simulink library "motohawk_engine_motoshare_lib"  (Simulink 6.3)
undefined symbols (not defined in the file or in its folder): cast_val, IndPowerMax, lookup_group, motohawk_tex, motohawk_vardec_config_group, motohawk_vardec_path, SampleTime, SteadyStateECT, txtTitle, WarmUpTimeConst
libraries: MotoHawk_lib x211, motohawk_control_primitives_lib x20, motohawk_annotations_lib x7, motohawk_engine_lib x5, AutoDoc_lib x4, motohawk_control_primitives_lib_new x3, motohawk_control_primitives_motoshare_lib x2
(part 2 of 7)

== system motohawk_engine_motoshare_lib/Discrete Actuator Characterization ==
  EngUnits : Inport
  0 = No Inversion 1 = Inversion : MotoHawk_lib/Calibration & Probing Blocks/motohawk_calibration  nam=[prefix '_Polarity']  val=boolean(polarity-1)  storage=Calibration  show_more=on  name_source=Use Parameter  data_type=Inherit from 'Default Value'  read_level=1  write_level=1  ovr_cals=on  view_as=Number  enum_struct={'Disabled', 'Enabled'}  vector_style=Wide Row  use_help_units=on  help="'Inverts the output of the actuator relative to the desired command - 0 = High True    1 = Low True'"  units='bool'  use_header_enum=off  row_header_enum={}  col_header_enum={}  use_min_max=off  min_val=-inf  max_val=inf  use_precision=off  precision=''  gain=1  offset=0  exp=1  use_mototune_group=on  mototune_group=[group ' | ' nam ' Config']
  Logical Operator : Logic  Operator=XOR
  Override in Engineering Units : MotoHawk_lib/Calibration & Probing Blocks/motohawk_override_abs  parent_name=prefix  show_more=on  name_source=Use Parameter  parent_read_level=1  parent_override_level=1  view_as=Number  enum_struct={'Disabled', 'Enabled'}  use_help_units=on  parent_help='Override actuator, in engineering units'  parent_units=units  use_min_max=off  parent_min=-inf  parent_max=inf  use_precision=off  parent_precision=''  parent_gain=1  parent_offset=0  parent_exp=1  use_mototune_group=on  parent_group=group
  Signal Specification : SignalSpecification  DataType=boolean
  motohawk_probe : MotoHawk_lib/Calibration & Probing Blocks/motohawk_probe  nam=prefix  show_more=on  name_source=Use Parameter  read_level=1  view_as=Number  enum_struct={'Disabled', 'Enabled'}  vector_style=Wide Row  use_help_units=on  help='Display output in engineering units'  units=units  use_header_enum=off  row_header_enum={}  col_header_enum={}  use_precision=off  precision=''  gain=1  offset=0  exp=1  use_mototune_group=on  mototune_group=group
  DiscOut : Outport
  wires:
  EngUnits/1 -> Signal Specification/1
  Signal Specification/1 -> Override in Engineering Units/1
  Override in Engineering Units/1 -> Logical Operator/1
  0 = No Inversion 1 = Inversion/1 -> Logical Operator/2
  Logical Operator/1 -> DiscOut/1, motohawk_probe/1

== system motohawk_engine_motoshare_lib/Engine Steady-State Flag ==
  Load : Inport
  RPM : Inport  Port=2
  Abs : Abs  SaturateOnIntegerOverflow=on
  Abs1 : Abs  SaturateOnIntegerOverflow=on
  Constant : Constant  Value=0
  Filter IndTorque : motohawk_control_primitives_lib/First Order Low Pass (Tunable)  nam='SSLoadFiltConst'  samp_time=samp_time  group=motohawk_vardec_config_group(group)
  Filter RPM : motohawk_control_primitives_lib/First Order Low Pass (Tunable)  nam='SSRPMFiltConst'  samp_time=samp_time  group=motohawk_vardec_config_group(group)
  Logical Operator : Logic  Inputs=3
  Relational Operator : RelationalOperator  Operator=<=  InputSameDT=on
  Relational Operator1 : RelationalOperator  Operator=<=  InputSameDT=on
  Relational Operator2 : RelationalOperator  Operator=>  ZeroCross=off  InputSameDT=on
  Steady-state RPM Tolerance [RPM] : MotoHawk_lib/Calibration & Probing Blocks/motohawk_calibration  nam='SSRPMTol'  val=500  storage=Calibration  show_more=on  name_source=Use Parameter  data_type=Inherit from 'Default Value'  read_level=1  write_level=1  ovr_cals=on  view_as=Number  enum_struct={'Disabled', 'Enabled'}  vector_style=Wide Row  use_help_units=on  help='Steady-State RPM Tolerance'  units='RPM'  use_header_enum=off  row_header_enum={}  col_header_enum={}  use_min_max=off  min_val=-inf  max_val=inf  use_precision=off  precision=''  gain=1  offset=0  exp=1  use_mototune_group=on  mototune_group=motohawk_vardec_config_group(group)
  Steady-state Torque Tolerance [N.m] : MotoHawk_lib/Calibration & Probing Blocks/motohawk_calibration  nam='SSLoadTol'  val=50  storage=Calibration  show_more=on  name_source=Use Parameter  data_type=Inherit from 'Default Value'  read_level=1  write_level=1  ovr_cals=on  view_as=Number  enum_struct={'Disabled', 'Enabled'}  vector_style=Wide Row  use_help_units=on  help='Steady-State Load Tolerance'  units=''  use_header_enum=off  row_header_enum={}  col_header_enum={}  use_min_max=off  min_val=-inf  max_val=inf  use_precision=off  precision=''  gain=1  offset=0  exp=1  use_mototune_group=on  mototune_group=motohawk_vardec_config_group(group)
  Sum : Sum  Inputs=+-|  SaturateOnIntegerOverflow=on  InputSameDT=on
  Sum1 : Sum  Inputs=+-|  SaturateOnIntegerOverflow=on  InputSameDT=on
  motohawk_probe : MotoHawk_lib/Calibration & Probing Blocks/motohawk_probe  nam='SSEngOpr'  show_more=on  name_source=Use Parameter  read_level=1  view_as=Enumeration  enum_struct={'Transient', 'Steady'}  vector_style=Wide Row  use_help_units=on  help='Steady-State Engine Operation'  units=''  use_header_enum=off  row_header_enum={}  col_header_enum={}  use_precision=off  precision=''  gain=1  offset=0  exp=1  use_mototune_group=on  mototune_group=group
  SSEngOpr [bool] : Outport
  wires:
  Constant/1 -> Relational Operator2/2
  Relational Operator2/1 -> Logical Operator/2
  Relational Operator/1 -> Logical Operator/3
  Relational Operator1/1 -> Logical Operator/1
  Load/1 -> Filter IndTorque/1, Sum/1
  RPM/1 -> Relational Operator2/1, Filter RPM/1, Sum1/1
  Filter IndTorque/1 -> Sum/2
  Sum/1 -> Abs/1
  Abs/1 -> Relational Operator/1
  Sum1/1 -> Abs1/1
  Abs1/1 -> Relational Operator1/1
  Logical Operator/1 -> motohawk_probe/1, SSEngOpr [bool]/1
  Filter RPM/1 -> Sum1/2
  Steady-state Torque Tolerance [N.m]/1 -> Relational Operator/2
  Steady-state RPM Tolerance [RPM]/1 -> Relational Operator1/2

== system motohawk_engine_motoshare_lib/Idle Governor ==
  RPM : Inport
  ECT [C] : Inport  Port=2
  ThrPos [%] : Inport  Port=3
  Idle State Determination : Subsystem
      mask Display: disp('IDLE STATE\nDETERMINATION');
  Logical Operator : Logic  Operator=NOT
  Ramp RPM : Subsystem
      mask Display: disp('RAMP RPM\nINTO IDLE STATE');
  Terminator3 : Terminator
  Universal PD (Tunable) : motohawk_control_primitives_lib/Universal PD (Tunable)  nam='Idle Spark Control'  prefix='IdleSpark_'  samp_time=SampleTime  units=''  group=motohawk_vardec_path(gcb)
  Universal PID (Tunable) : motohawk_control_primitives_lib/Universal PID (Tunable)  nam='Idle Air Control'  prefix='IdleAir_'  samp_time=SampleTime  units=''  group=motohawk_vardec_path(gcb)
  motohawk_calibration2 : MotoHawk_lib/Calibration & Probing Blocks/motohawk_calibration  nam='IdleTargetRPM'  val=500  storage=Calibration  show_more=on  name_source=Use Parameter  data_type=Inherit from 'Default Value'  read_level=1  write_level=1  ovr_cals=on  view_as=Number  enum_struct={'Disabled', 'Enabled'}  vector_style=Wide Row  use_help_units=off  help=''  units=''  use_header_enum=off  row_header_enum={}  col_header_enum={}  use_min_max=off  min_val=-inf  max_val=inf  use_precision=off  precision=''  gain=1  offset=0  exp=1  use_mototune_group=off  mototune_group=motohawk_vardec_path(gcb)
  SparkAdv Offset [degCA] : Outport
  LIAC Offset [%] : Outport  Port=2
  wires:
  Logical Operator/1 -> Universal PID (Tunable)/3
  motohawk_calibration2/1 -> Ramp RPM/3(TargetRPM), Idle State Determination/2(TargetRPM)
  Universal PID (Tunable)/1 -> LIAC Offset [%]/1
  Idle State Determination/1(OnIdle) -> Logical Operator/1, Ramp RPM/1(OnIdle)
  Ramp RPM/1(RPMSetPt) -> Universal PD (Tunable)/2, Universal PID (Tunable)/2  "RPMSetPt"
  Universal PD (Tunable)/1 -> SparkAdv Offset [degCA]/1
  ThrPos [%]/1 -> Idle State Determination/3(ThrPos [%])
  RPM/1 -> Universal PID (Tunable)/1, Universal PD (Tunable)/1, Ramp RPM/2(RPM), Idle State Determination/1(RPM)  "RPM"
  ECT [C]/1 -> Terminator3/1

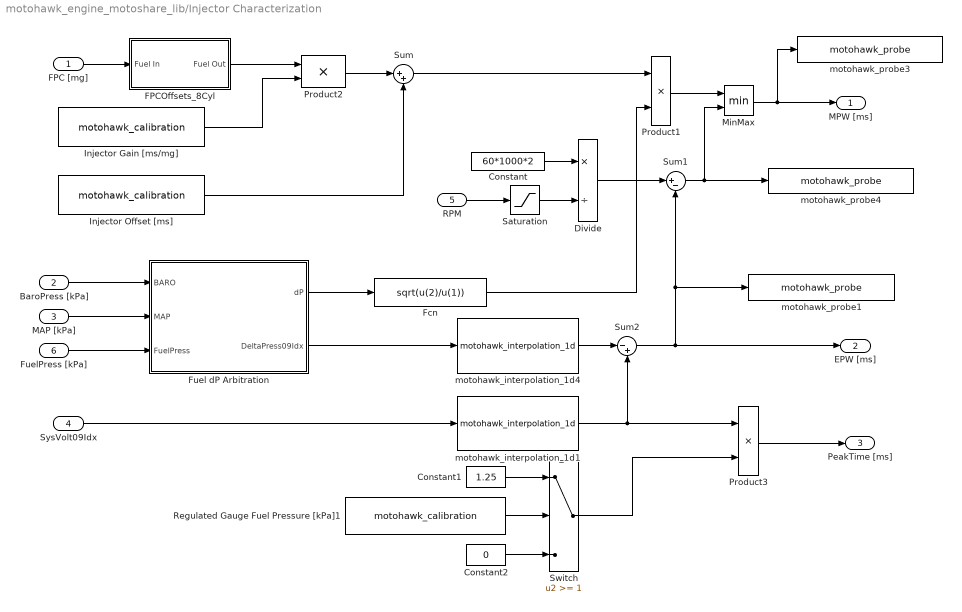
== system motohawk_engine_motoshare_lib/Injector Characterization ==
  FPC [mg] : Inport
  BaroPress [kPa] : Inport  Port=2
  MAP [kPa] : Inport  Port=3
  SysVolt09Idx : Inport  Port=4
  RPM : Inport  Port=5
  FuelPress [kPa] : Inport  Port=6
  Constant : Constant  Value=60*1000*2
  Constant1 : Constant  Value=1.25
  Constant2 : Constant  Value=0
  Divide : Product  Inputs=*/  OutScaling=2^-10
  FPCOffsets_8Cyl : Subsystem
  Fcn : Fcn  Expr=sqrt(u(2)/u(1))
  Fuel dP Arbitration : Subsystem
  Injector Gain [ms/mg] : MotoHawk_lib/Calibration & Probing Blocks/motohawk_calibration  nam='InjGain'  val=0.351  storage=Calibration  show_more=on  name_source=Use Parameter  data_type=Inherit from 'Default Value'  read_level=1  write_level=1  ovr_cals=on  view_as=Number  enum_struct={'Disabled', 'Enabled'}  vector_style=Wide Row  use_help_units=on  help='Gain value used in the linear transformation of FPC to mechanical pulsewidth.'  units='ms/mg'  use_header_enum=off  row_header_enum={}  col_header_enum={}  use_min_max=off  min_val=0  max_val=inf  use_precision=off  precision='2.4'  gain=1  offset=0  exp=1  use_mototune_group=on  mototune_group='Actuators | Injectors | Injector Config'
  Injector Offset [ms] : MotoHawk_lib/Calibration & Probing Blocks/motohawk_calibration  nam='InjOffset'  val=-0.05  storage=Calibration  show_more=on  name_source=Use Parameter  data_type=Inherit from 'Default Value'  read_level=1  write_level=1  ovr_cals=on  view_as=Number  enum_struct={'Disabled', 'Enabled'}  vector_style=Wide Row  use_help_units=on  help='Offset value used in the linear transformation of FPC to mechanical pulsewidth.'  units='ms'  use_header_enum=off  row_header_enum={}  col_header_enum={}  use_min_max=off  min_val=-inf  max_val=inf  use_precision=off  precision='3.4'  gain=1  offset=0  exp=1  use_mototune_group=on  mototune_group='Actuators | Injectors | Injector Config'
  MinMax : MinMax  Inputs=2
  Product1 : Product  SaturateOnIntegerOverflow=on  InputSameDT=on
  Product2 : Product  SaturateOnIntegerOverflow=on  InputSameDT=on
  Product3 : Product  SaturateOnIntegerOverflow=on  InputSameDT=on
  Regulated Gauge Fuel Pressure [kPa]1 : MotoHawk_lib/Calibration & Probing Blocks/motohawk_calibration  nam='InjectorType'  val=0  storage=Calibration  show_more=on  name_source=Use Parameter  data_type=int8  read_level=1  write_level=1  ovr_cals=on  view_as=Enumeration  enum_struct={'HighImpedance', 'LowImpedance'}  vector_style=Wide Row  use_help_units=on  help='Selects whether to use the peak and hold feature of the fuel injector driver.'  units=''  use_header_enum=off  row_header_enum={}  col_header_enum={}  use_min_max=on  min_val=-inf  max_val=inf  use_precision=off  precision=''  gain=1  offset=0  exp=1  use_mototune_group=on  mototune_group='Actuators | Injectors | Injector Config'
  Saturation : Saturate  UpperLimit=inf  LowerLimit=.01
  Sum : Sum  Inputs=|++  SaturateOnIntegerOverflow=on  InputSameDT=on
  Sum1 : Sum  Inputs=|+-  SaturateOnIntegerOverflow=on
  Sum2 : Sum  Inputs=|-+  SaturateOnIntegerOverflow=on
  Switch : Switch  Threshold=1
  motohawk_interpolation_1d1 : MotoHawk_lib/Lookup Tables/motohawk_interpolation_1d  nam='InjTurnOn'  table_data=zeros(1,9)  show_more=on  data_type=Inherit from 'Table Data'  storage=NonAdaptive  read_level=1  write_level=1  ovr_cals=on  use_help=on  help='Injector turn on time.'  units='ms'  use_min_max=off  min_val=-inf  max_val=inf  use_precision=off  precision='2.3'  gain=1  offset=0  exp=1  use_links=off  prelookup_block=''  output_name=''  use_mototune_group=on  mototune_group='Actuators | Injectors'
  motohawk_interpolation_1d4 : MotoHawk_lib/Lookup Tables/motohawk_interpolation_1d  nam='InjTurnOff'  table_data=zeros(1,9)  show_more=on  data_type=Inherit from 'Table Data'  storage=NonAdaptive  read_level=1  write_level=1  ovr_cals=on  use_help=on  help='Injector turn off time'  units='ms'  use_min_max=on  min_val=-inf  max_val=inf  use_precision=on  precision='2.3'  gain=1  offset=0  exp=1  use_links=off  prelookup_block=''  output_name=''  use_mototune_group=on  mototune_group='Actuators | Injectors'
  motohawk_probe1 : MotoHawk_lib/Calibration & Probing Blocks/motohawk_probe  nam='InjEPW'  show_more=on  name_source=Use Parameter  read_level=1  view_as=Number  enum_struct={'Disabled', 'Enabled'}  vector_style=Wide Row  use_help_units=on  help=''  units=''  use_header_enum=off  row_header_enum={}  col_header_enum={}  use_precision=off  precision=''  gain=1  offset=0  exp=1  use_mototune_group=on  mototune_group='Actuators | Injectors'
  motohawk_probe3 : MotoHawk_lib/Calibration & Probing Blocks/motohawk_probe  nam='InjMPW'  show_more=on  name_source=Use Parameter  read_level=1  view_as=Number  enum_struct={'Disabled', 'Enabled'}  vector_style=Wide Row  use_help_units=on  help=''  units=''  use_header_enum=off  row_header_enum={}  col_header_enum={}  use_precision=off  precision=''  gain=1  offset=0  exp=1  use_mototune_group=on  mototune_group='Actuators | Injectors'
  motohawk_probe4 : MotoHawk_lib/Calibration & Probing Blocks/motohawk_probe  nam='MaxAllowableMPW'  show_more=on  name_source=Use Parameter  read_level=1  view_as=Number  enum_struct={'Disabled', 'Enabled'}  vector_style=Wide Row  use_help_units=on  help=''  units=''  use_header_enum=off  row_header_enum={}  col_header_enum={}  use_precision=off  precision=''  gain=1  offset=0  exp=1  use_mototune_group=on  mototune_group='Actuators | Injectors'
  MPW [ms] : Outport
  EPW [ms] : Outport  Port=2
  PeakTime [ms] : Outport  Port=3
  wires:
  Fcn/1 -> Product1/2
  Saturation/1 -> Divide/2
  RPM/1 -> Saturation/1
  Divide/1 -> Sum1/1
  Sum1/1 -> motohawk_probe4/1, MinMax/2
  MinMax/1 -> MPW [ms]/1, motohawk_probe3/1
  Product1/1 -> MinMax/1
  Constant/1 -> Divide/1
  Product2/1 -> Sum/1
  Sum2/1 -> motohawk_probe1/1, Sum1/2, EPW [ms]/1
  motohawk_interpolation_1d4/1 -> Sum2/1
  motohawk_interpolation_1d1/1 -> Sum2/2, Product3/1
  Sum/1 -> Product1/1
  SysVolt09Idx/1 -> motohawk_interpolation_1d1/1
  Injector Offset [ms]/1 -> Sum/2
  Injector Gain [ms/mg]/1 -> Product2/2
  FPC [mg]/1 -> FPCOffsets_8Cyl/1(Fuel In)
  Product3/1 -> PeakTime [ms]/1
  Regulated Gauge Fuel Pressure [kPa]1/1 -> Switch/2
  Constant1/1 -> Switch/1
  Constant2/1 -> Switch/3
  Switch/1 -> Product3/2
  BaroPress [kPa]/1 -> Fuel dP Arbitration/1(BARO)
  MAP [kPa]/1 -> Fuel dP Arbitration/2(MAP)
  FuelPress [kPa]/1 -> Fuel dP Arbitration/3(FuelPress)
  Fuel dP Arbitration/2(DeltaPress09Idx) -> motohawk_interpolation_1d4/1
  Fuel dP Arbitration/1(dP) -> Fcn/1
  FPCOffsets_8Cyl/1(Fuel Out) -> Product2/1

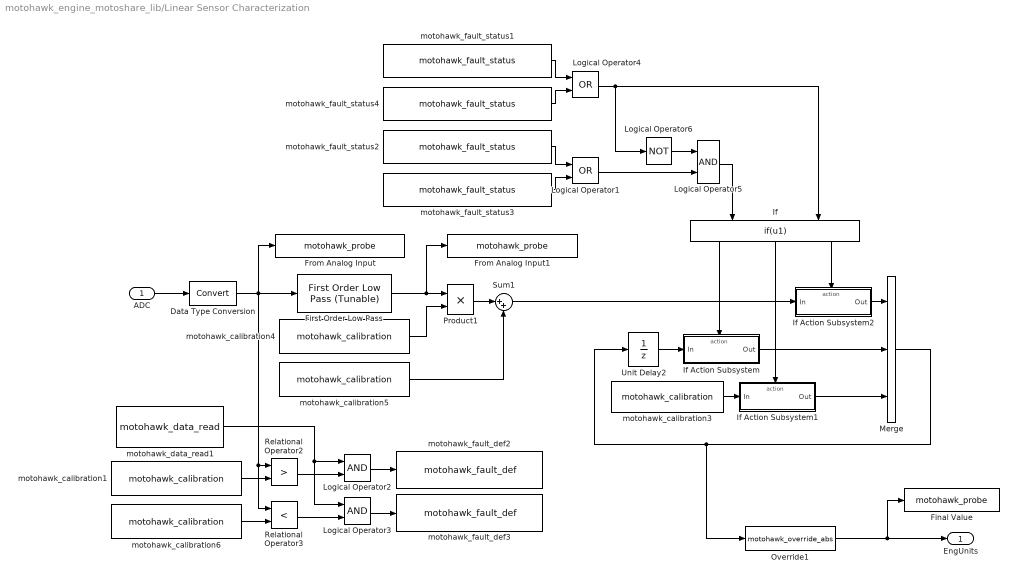
== system motohawk_engine_motoshare_lib/Linear Sensor Characterization ==
  ADC : Inport
  Data Type Conversion : DataTypeConversion  SaturateOnIntegerOverflow=on  RndMeth=Zero
  Final Value : MotoHawk_lib/Calibration & Probing Blocks/motohawk_probe  nam=[prefix]  show_more=on  name_source=Use Parameter  read_level=1  view_as=Number  enum_struct={'Disabled', 'Enabled'}  vector_style=Wide Row  use_help_units=on  help='Final value after Linear Sensor Characterization'  units=units  use_header_enum=off  row_header_enum={}  col_header_enum={}  use_precision=off  precision=''  gain=1  offset=0  exp=1  use_mototune_group=on  mototune_group=group
  First Order Low Pass : motohawk_control_primitives_lib/First Order Low Pass (Tunable)  nam=[prefix 'FilterConst']  samp_time=samp_time  group=[group ' | ' nam ' Config']
  From Analog Input : MotoHawk_lib/Calibration & Probing Blocks/motohawk_probe  nam=[prefix 'ADCRaw']  show_more=on  name_source=Use Parameter  read_level=1  view_as=Number  enum_struct={'Disabled', 'Enabled'}  vector_style=Wide Row  use_help_units=on  help='Singal measured directly from sensor'  units=inputunits  use_header_enum=off  row_header_enum={}  col_header_enum={}  use_precision=off  precision=''  gain=1  offset=0  exp=1  use_mototune_group=on  mototune_group=group
  From Analog Input1 : MotoHawk_lib/Calibration & Probing Blocks/motohawk_probe  nam=[prefix 'ADCFilt']  show_more=on  name_source=Use Parameter  read_level=1  view_as=Number  enum_struct={'Disabled', 'Enabled'}  vector_style=Wide Row  use_help_units=on  help='Singal measured directly from sensor'  units=inputunits  use_header_enum=off  row_header_enum={}  col_header_enum={}  use_precision=off  precision=''  gain=1  offset=0  exp=1  use_mototune_group=on  mototune_group=group
  If : If  Orientation=down  NumInputs=2  IfExpression=u1  ElseIfExpressions=u2  ZeroCross=off
  If Action Subsystem : Subsystem  TreatAsAtomicUnit=on
      mask Display: disp('Saturate');
  If Action Subsystem1 : Subsystem  TreatAsAtomicUnit=on
      mask Display: disp('Default');
  If Action Subsystem2 : Subsystem  TreatAsAtomicUnit=on
      mask Display: disp('Pass Through');
  Logical Operator1 : Logic  Operator=OR
  Logical Operator2 : Logic
  Logical Operator3 : Logic
  Logical Operator4 : Logic  Operator=OR
  Logical Operator5 : Logic
  Logical Operator6 : Logic  Operator=NOT
  Merge : Merge  Inputs=3
  Override1 : MotoHawk_lib/Calibration & Probing Blocks/motohawk_override_abs  parent_name=nam  show_more=on  name_source=Use Parameter  parent_read_level=1  parent_override_level=1  view_as=Number  enum_struct={'Disabled', 'Enabled'}  use_help_units=on  parent_help='Override result of linear sensor characterization, in engineering units'  parent_units=units  use_min_max=on  parent_min=-inf  parent_max=inf  use_precision=off  parent_precision=''  parent_gain=1  parent_offset=0  parent_exp=1  use_mototune_group=on  parent_group=group
  Product1 : Product  SaturateOnIntegerOverflow=on  InputSameDT=on
  Relational Operator2 : RelationalOperator  Operator=>  ZeroCross=off  InputSameDT=on
  Relational Operator3 : RelationalOperator  Operator=<  ZeroCross=off  InputSameDT=on
  Sum1 : Sum  Inputs=|++  SaturateOnIntegerOverflow=on
  Unit Delay2 : UnitDelay  SampleTime=-1
  motohawk_calibration1 : MotoHawk_lib/Calibration & Probing Blocks/motohawk_calibration  nam=[prefix 'RangeHiLimit']  val=1013  storage=Calibration  show_more=on  name_source=Use Parameter  data_type=double  read_level=1  write_level=1  ovr_cals=on  view_as=Number  enum_struct={'Disabled', 'Enabled'}  vector_style=Wide Row  use_help_units=on  help='Maximum allowable input, indicating short or open circuit'  units=inputunits  use_header_enum=off  row_header_enum={}  col_header_enum={}  use_min_max=off  min_val=-inf  max_val=inf  use_precision=off  precision=''  gain=1  offset=0  exp=1  use_mototune_group=on  mototune_group=[group ' | ' nam ' Config']
  motohawk_calibration3 : MotoHawk_lib/Calibration & Probing Blocks/motohawk_calibration  nam=[prefix 'DfltValue']  val=1  storage=Calibration  show_more=on  name_source=Use Parameter  data_type=double  read_level=1  write_level=1  ovr_cals=on  view_as=Number  enum_struct={'Disabled', 'Enabled'}  vector_style=Wide Row  use_help_units=on  help="'This is the initial default value should the sensor be in fault on key-up.  Otherwise the sensors outputs the last value prior to faulting'"  units=units  use_header_enum=off  row_header_enum={}  col_header_enum={}  use_min_max=off  min_val=-inf  max_val=inf  use_precision=off  precision=''  gain=1  offset=0  exp=1  use_mototune_group=on  mototune_group=[group ' | ' nam ' Config']
  motohawk_calibration4 : MotoHawk_lib/Calibration & Probing Blocks/motohawk_calibration  nam=[prefix 'Gain']  val=1  storage=Calibration  show_more=on  name_source=Use Parameter  data_type=double  read_level=1  write_level=1  ovr_cals=on  view_as=Number  enum_struct={'Disabled', 'Enabled'}  vector_style=Wide Row  use_help_units=on  help='Scaling from A/D counts to engineering units'  units=[units '/ADC']  use_header_enum=off  row_header_enum={}  col_header_enum={}  use_min_max=off  min_val=-inf  max_val=inf  use_precision=on  precision='5.4'  gain=1  offset=0  exp=1  use_mototune_group=on  mototune_group=[group ' | ' nam ' Config']
  motohawk_calibration5 : MotoHawk_lib/Calibration & Probing Blocks/motohawk_calibration  nam=[prefix 'Ofst']  val=0  storage=Calibration  show_more=on  name_source=Use Parameter  data_type=double  read_level=1  write_level=1  ovr_cals=on  view_as=Number  enum_struct={'Disabled', 'Enabled'}  vector_style=Wide Row  use_help_units=on  help='Offset after gain in engineering units'  units=units  use_header_enum=off  row_header_enum={}  col_header_enum={}  use_min_max=off  min_val=-inf  max_val=inf  use_precision=off  precision=''  gain=1  offset=0  exp=1  use_mototune_group=on  mototune_group=[group ' | ' nam ' Config']
  motohawk_calibration6 : MotoHawk_lib/Calibration & Probing Blocks/motohawk_calibration  nam=[prefix 'RangeLoLimit']  val=10  storage=Calibration  show_more=on  name_source=Use Parameter  data_type=double  read_level=1  write_level=1  ovr_cals=on  view_as=Number  enum_struct={'Disabled', 'Enabled'}  vector_style=Wide Row  use_help_units=on  help='Minimum allowable input, indicating short or open circuit'  units=inputunits  use_header_enum=off  row_header_enum={}  col_header_enum={}  use_min_max=off  min_val=-inf  max_val=inf  use_precision=off  precision=''  gain=1  offset=0  exp=1  use_mototune_group=on  mototune_group=[group ' | ' nam ' Config']
  motohawk_data_read1 : MotoHawk_lib/Data Storage Blocks/motohawk_data_read  source=Lookup By Name  structure=Scalar  operation=Read entire data structure at once  sz_vec=4  sz_row=2  sz_col=3  typ=boolean  nam='MPRD'  checkNull=on  struct_inst_name='Struct1'
  motohawk_fault_def2 : MotoHawk_lib/Fault Management Blocks/motohawk_fault_def  nam=[prefix 'RangeHi']  mode=Enabled  id=[]  x=25  y=50  input_suspected=on  indeterminate=off  increment_xy=on  downsample_count=1  ovr_cals=on  ovr_actions=on  show_actions=off  action1_name=''  action1_cond=(None)  action2_name=''  action2_cond=(None)  action3_name=''  action3_cond=(None)  action4_name=''  action4_cond=(None)
  motohawk_fault_def3 : MotoHawk_lib/Fault Management Blocks/motohawk_fault_def  nam=[prefix 'RangeLo']  mode=Enabled  id=[]  x=25  y=50  input_suspected=on  indeterminate=off  increment_xy=on  downsample_count=1  ovr_cals=on  ovr_actions=on  show_actions=off  action1_name=''  action1_cond=(None)  action2_name=''  action2_cond=(None)  action3_name=''  action3_cond=(None)  action4_name=''  action4_cond=(None)
  motohawk_fault_status1 : MotoHawk_lib/Fault Management Blocks/motohawk_fault_status  source=Lookup By Name  nam=[prefix 'RangeHigh']  status=Active
  motohawk_fault_status2 : MotoHawk_lib/Fault Management Blocks/motohawk_fault_status  source=Lookup By Name  nam=[prefix 'RangeHigh']  status=Suspected
  motohawk_fault_status3 : MotoHawk_lib/Fault Management Blocks/motohawk_fault_status  source=Lookup By Name  nam=[prefix 'RangeLow']  status=Suspected
  motohawk_fault_status4 : MotoHawk_lib/Fault Management Blocks/motohawk_fault_status  source=Lookup By Name  nam=[prefix 'RangeLow']  status=Active
  EngUnits : Outport
  wires:
  Merge/1 -> Override1/1, Unit Delay2/1
  If/3 -> If Action Subsystem2/Action
  If/1 -> If Action Subsystem/Action
  Data Type Conversion/1 -> Relational Operator2/1, Relational Operator3/1, First Order Low Pass/1, From Analog Input/1
  ADC/1 -> Data Type Conversion/1
  motohawk_calibration4/1 -> Product1/2
  motohawk_calibration5/1 -> Sum1/2
  Product1/1 -> Sum1/1
  motohawk_data_read1/1 -> Logical Operator2/1, Logical Operator3/1
  Logical Operator3/1 -> motohawk_fault_def3/1
  Logical Operator2/1 -> motohawk_fault_def2/1
  Relational Operator3/1 -> Logical Operator3/2
  Relational Operator2/1 -> Logical Operator2/2
  motohawk_calibration1/1 -> Relational Operator2/2
  motohawk_calibration6/1 -> Relational Operator3/2
  motohawk_fault_status2/1 -> Logical Operator1/1
  motohawk_fault_status3/1 -> Logical Operator1/2
  If Action Subsystem2/1(Out) -> Merge/1
  If Action Subsystem/1(Out) -> Merge/2
  Sum1/1 -> If Action Subsystem2/1(In)
  motohawk_fault_status1/1 -> Logical Operator4/1
  motohawk_fault_status4/1 -> Logical Operator4/2
  If Action Subsystem1/1(Out) -> Merge/3
  If/2 -> If Action Subsystem1/Action
  motohawk_calibration3/1 -> If Action Subsystem1/1(In)
  Logical Operator6/1 -> Logical Operator5/1
  Logical Operator5/1 -> If/1
  Logical Operator1/1 -> Logical Operator5/2
  Logical Operator4/1 -> Logical Operator6/1, If/2
  Override1/1 -> Final Value/1, EngUnits/1
  Unit Delay2/1 -> If Action Subsystem/1(In)
  First Order Low Pass/1 -> Product1/1, From Analog Input1/1

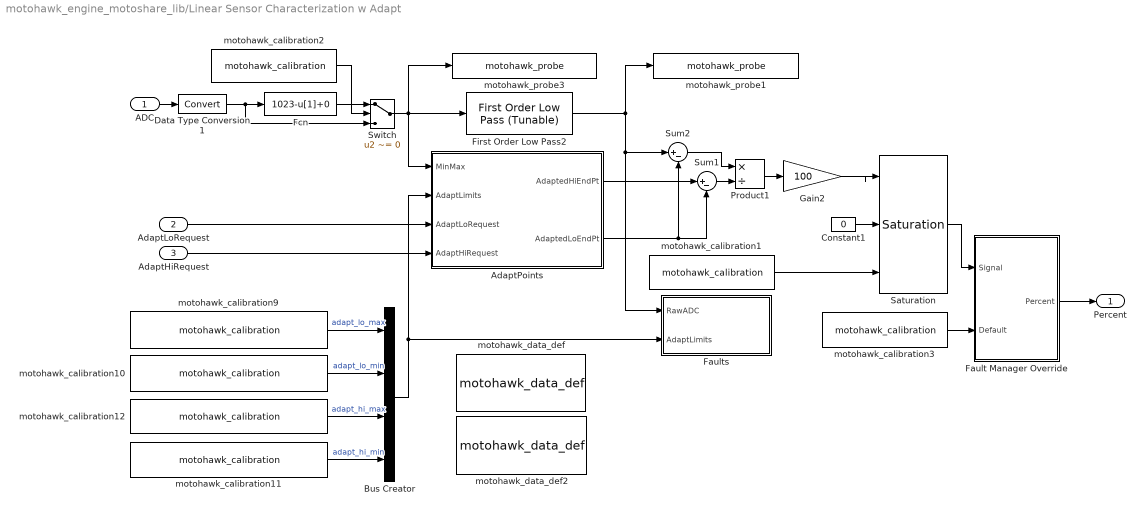
== system motohawk_engine_motoshare_lib/Linear Sensor Characterization w Adapt ==
  ADC : Inport
  AdaptLoRequest : Inport  Port=2
  AdaptHiRequest : Inport  Port=3
  AdaptPoints : Subsystem
  Bus Creator : BusCreator
  Constant1 : Constant  Value=0  OutDataTypeMode=double
  Data Type Conversion1 : DataTypeConversion  OutDataTypeMode=double  SaturateOnIntegerOverflow=on  RndMeth=Zero
  Fault Manager Override : Subsystem
  Faults : Subsystem
  Fcn : Fcn  Expr=1023-u[1]+0
  First Order Low Pass2 : motohawk_control_primitives_lib/First Order Low Pass (Tunable)  nam=[prefix 'FilterConst']  samp_time=samp_time  group=[group ' | ' nam ' Config']
  Gain2 : Gain  Gain=100  SaturateOnIntegerOverflow=on
  Product1 : Product  Inputs=*/  SaturateOnIntegerOverflow=on  InputSameDT=on
  Saturation : motohawk_control_primitives_lib/Saturation
  Sum1 : Sum  Inputs=|+-  SaturateOnIntegerOverflow=on
  Sum2 : Sum  Inputs=|+-  SaturateOnIntegerOverflow=on
  Switch : Switch  Criteria=u2 ~= 0  SaturateOnIntegerOverflow=on
  motohawk_calibration1 : MotoHawk_lib/Calibration & Probing Blocks/motohawk_calibration  nam=[prefix 'MaxLimit']  val=100  storage=Calibration  show_more=on  name_source=Use Parameter  data_type=double  read_level=1  write_level=1  ovr_cals=on  view_as=Number  enum_struct={'Disabled', 'Enabled'}  vector_style=Wide Row  use_help_units=on  help='Sets the upper limit on the potentiometer range.'  units=units  use_header_enum=off  row_header_enum={}  col_header_enum={}  use_min_max=off  min_val=-inf  max_val=inf  use_precision=off  precision=''  gain=1  offset=0  exp=1  use_mototune_group=on  mototune_group=[group ' | ' nam ' Config']
  motohawk_calibration10 : MotoHawk_lib/Calibration & Probing Blocks/motohawk_calibration  nam=[prefix 'AdaptLowMin']  val=100  storage=Calibration  show_more=on  name_source=Use Parameter  data_type=Inherit from 'Default Value'  read_level=1  write_level=1  ovr_cals=on  view_as=Number  enum_struct={'Disabled', 'Enabled'}  vector_style=Wide Row  use_help_units=on  help='Specifies for the minimum value of the lower adapt range.'  units='ADC Counts'  use_header_enum=off  row_header_enum={}  col_header_enum={}  use_min_max=off  min_val=-inf  max_val=inf  use_precision=off  precision=''  gain=1  offset=0  exp=1  use_mototune_group=on  mototune_group=[group ' | ' nam ' Config']
  motohawk_calibration11 : MotoHawk_lib/Calibration & Probing Blocks/motohawk_calibration  nam=[prefix 'AdaptHiMin']  val=700  storage=Calibration  show_more=on  name_source=Use Parameter  data_type=Inherit from 'Default Value'  read_level=1  write_level=1  ovr_cals=on  view_as=Number  enum_struct={'Disabled', 'Enabled'}  vector_style=Wide Row  use_help_units=on  help='Specifies for the minimum value of the upper adapt range.'  units='ADC Counts'  use_header_enum=off  row_header_enum={}  col_header_enum={}  use_min_max=off  min_val=-inf  max_val=inf  use_precision=off  precision=''  gain=1  offset=0  exp=1  use_mototune_group=on  mototune_group=[group ' | ' nam ' Config']
  motohawk_calibration12 : MotoHawk_lib/Calibration & Probing Blocks/motohawk_calibration  nam=[prefix 'AdaptHiMax']  val=900  storage=Calibration  show_more=on  name_source=Use Parameter  data_type=Inherit from 'Default Value'  read_level=1  write_level=1  ovr_cals=on  view_as=Number  enum_struct={'Disabled', 'Enabled'}  vector_style=Wide Row  use_help_units=on  help='Specifies for the maximum value of the upper adapt range.'  units='ADC Counts'  use_header_enum=off  row_header_enum={}  col_header_enum={}  use_min_max=off  min_val=-inf  max_val=inf  use_precision=off  precision=''  gain=1  offset=0  exp=1  use_mototune_group=on  mototune_group=[group ' | ' nam ' Config']
  motohawk_calibration2 : MotoHawk_lib/Calibration & Probing Blocks/motohawk_calibration  nam=[prefix 'Rev_Polarity']  val=false  storage=Calibration  show_more=on  name_source=Use Parameter  data_type=boolean  read_level=1  write_level=1  ovr_cals=on  view_as=Number  enum_struct={'Disabled', 'Enabled'}  vector_style=Wide Row  use_help_units=on  help='1 = Reverse Polarity (Smaller voltage values indicate larger % travel)'  units='boolean'  use_header_enum=off  row_header_enum={}  col_header_enum={}  use_min_max=off  min_val=-inf  max_val=inf  use_precision=off  precision=''  gain=1  offset=0  exp=1  use_mototune_group=on  mototune_group=[group ' | ' nam ' Config']
  motohawk_calibration3 : MotoHawk_lib/Calibration & Probing Blocks/motohawk_calibration  nam=[prefix 'DfltValue']  val=10  storage=Calibration  show_more=on  name_source=Use Parameter  data_type=double  read_level=1  write_level=1  ovr_cals=on  view_as=Number  enum_struct={'Disabled', 'Enabled'}  vector_style=Wide Row  use_help_units=on  help="'This is the initial default value should the sensor be in fault on key-up.  Otherwise the sensors outputs the last value prior to faulting'"  units=units  use_header_enum=off  row_header_enum={}  col_header_enum={}  use_min_max=off  min_val=-inf  max_val=inf  use_precision=off  precision=''  gain=1  offset=0  exp=1  use_mototune_group=on  mototune_group=[group ' | ' nam ' Config']
  motohawk_calibration9 : MotoHawk_lib/Calibration & Probing Blocks/motohawk_calibration  nam=[prefix 'AdaptLowMax']  val=300  storage=Calibration  show_more=on  name_source=Use Parameter  data_type=Inherit from 'Default Value'  read_level=1  write_level=1  ovr_cals=on  view_as=Number  enum_struct={'Disabled', 'Enabled'}  vector_style=Wide Row  use_help_units=on  help='Specifies for the maximum value of the lower adapt range.'  units='ADC Counts'  use_header_enum=off  row_header_enum={}  col_header_enum={}  use_min_max=off  min_val=-inf  max_val=inf  use_precision=off  precision=''  gain=1  offset=0  exp=1  use_mototune_group=on  mototune_group=[group ' | ' nam ' Config']
  motohawk_data_def : MotoHawk_lib/Data Storage Blocks/motohawk_data_def  nam=[prefix 'RawAdptLow']  data=499  typ=uint16  struct_nam='MyStruct'  storage=NonVolatile  outputRef=off  use_vardec=off  window=Calibration  read_level=1  write_level=1  ovr_cals=on  view_as=Number  enum_struct={'Disabled', 'Enabled'}  vector_style=Wide Row  use_help_units=off  help=''  units=''  use_header_enum=off  row_header_enum={}  col_header_enum={}  use_min_max=off  min_val=-inf  max_val=inf  use_precision=off  precision=''  gain=1  offset=0  exp=1  use_mototune_group=off  mototune_group=motohawk_vardec_path(gcb)  eval_name=TPSRawAdptLow
  motohawk_data_def2 : MotoHawk_lib/Data Storage Blocks/motohawk_data_def  nam=[prefix 'RawAdptHi']  data=500  typ=uint16  struct_nam='MyStruct'  storage=NonVolatile  outputRef=off  use_vardec=off  window=Calibration  read_level=1  write_level=1  ovr_cals=on  view_as=Number  enum_struct={'Disabled', 'Enabled'}  vector_style=Wide Row  use_help_units=off  help=''  units=''  use_header_enum=off  row_header_enum={}  col_header_enum={}  use_min_max=off  min_val=-inf  max_val=inf  use_precision=off  precision=''  gain=1  offset=0  exp=1  use_mototune_group=off  mototune_group=motohawk_vardec_path(gcb)  eval_name=TPSRawAdptHi
  motohawk_probe1 : MotoHawk_lib/Calibration & Probing Blocks/motohawk_probe  nam=[prefix 'ADCFilt']  show_more=on  name_source=Use Parameter  read_level=1  view_as=Number  enum_struct={'Disabled', 'Enabled'}  vector_style=Wide Row  use_help_units=on  help=''  units=''  use_header_enum=off  row_header_enum={}  col_header_enum={}  use_precision=on  precision=''  gain=1  offset=0  exp=1  use_mototune_group=on  mototune_group=group
  motohawk_probe3 : MotoHawk_lib/Calibration & Probing Blocks/motohawk_probe  nam=[prefix 'ADCRaw']  show_more=on  name_source=Use Parameter  read_level=1  view_as=Number  enum_struct={'Disabled', 'Enabled'}  vector_style=Wide Row  use_help_units=on  help=''  units=''  use_header_enum=off  row_header_enum={}  col_header_enum={}  use_precision=on  precision=''  gain=1  offset=0  exp=1  use_mototune_group=on  mototune_group=group
  Percent : Outport
  wires:
  motohawk_calibration3/1 -> Fault Manager Override/2(Default)
  Saturation/1 -> Fault Manager Override/1(Signal)
  Fault Manager Override/1(Percent) -> Percent/1
  motohawk_calibration1/1 -> Saturation/3
  Gain2/1 -> Saturation/1
  Switch/1 -> AdaptPoints/1(MinMax), motohawk_probe3/1, First Order Low Pass2/1
  motohawk_calibration2/1 -> Switch/2
  Fcn/1 -> Switch/1
  Data Type Conversion1/1 -> Switch/3, Fcn/1
  ADC/1 -> Data Type Conversion1/1
  Bus Creator/1 -> Faults/2(AdaptLimits), AdaptPoints/2(AdaptLimits)
  motohawk_calibration11/1 -> Bus Creator/4  "adapt_hi_min"
  motohawk_calibration12/1 -> Bus Creator/3  "adapt_hi_max"
  motohawk_calibration10/1 -> Bus Creator/2  "adapt_lo_min"
  motohawk_calibration9/1 -> Bus Creator/1  "adapt_lo_max"
  Sum1/1 -> Product1/2
  Product1/1 -> Gain2/1
  Sum2/1 -> Product1/1
  Constant1/1 -> Saturation/2
  AdaptPoints/2(AdaptedLoEndPt) -> Sum1/2, Sum2/2
  AdaptPoints/1(AdaptedHiEndPt) -> Sum1/1
  AdaptLoRequest/1 -> AdaptPoints/3(AdaptLoRequest)
  AdaptHiRequest/1 -> AdaptPoints/4(AdaptHiRequest)
  First Order Low Pass2/1 -> Faults/1(RawADC), Sum2/1, motohawk_probe1/1

== system motohawk_engine_motoshare_lib/Load, Torque, Power, Work - Using APC ==
  note: Lookup Load and Torque
  MAF [g/s] : Inport
  RPM : Inport  Port=2
  EventsPerRev : Inport  Port=3
  Air Per Cylinder Calculation : motohawk_engine_lib/Mass Flow to Charge Mass Transform
  Calculate Power and Work : Subsystem
  motohawk_TitleBlock : motohawk_annotations_lib/motohawk_TitleBlock  BlockType_='Mototron_Title_Block'  ttl='Calculate Observed Engine States, such as Load, Torque, and Power\newline\rmUsing Airflow rate, calculate Air per Cylinder, and lookup Load and Torque values.'  copyright="'THE INFORMATION CONTAINED IN THIS\\newlineDRAWING IS THE SOLE PROPERTY OF\\newlineMOTOTRON.  ANY REPRODUCTION IN\\newline PART OR AS A WHOLE WITHOUT THE\\newlineWRITTEN PERMISSION OF MOTOTRON\\newline IS PROHIBITED.\\fontsize{16}\\rm\\copyright\\rm\\fontsize{10} 2005'"  address='\fontsize{22}\it\fontname{Arial Black}MotoTron Corporation \fontname{Arial}\fontsize{10}\newline505 Marion Road, Oshkosh, WI, 54901\newlinewww.mototron.com (734) 822-7700'  image_file='mh.jpg'  pretty_print=on  edit_text=[motohawk_tex(get_param(bdroot, 'Description')) '\rm\newline' motohawk_tex(get_param(gcs, 'Name'))]  edit_as=6
  motohawk_probe : MotoHawk_lib/Calibration & Probing Blocks/motohawk_probe  nam='APC'  show_more=on  name_source=Use Parameter  read_level=1  view_as=Number  enum_struct={'Disabled', 'Enabled'}  vector_style=Wide Row  use_help_units=on  help='Air Per Cylinder - Calculated from MAF model'  units='mg'  use_header_enum=off  row_header_enum={}  col_header_enum={}  use_precision=off  precision=''  gain=1  offset=0  exp=1  use_mototune_group=off  mototune_group=lookup_group(gcb, 'APC')
  motohawk_table_1d : MotoHawk_lib/Lookup Tables/motohawk_table_1d  nam='IndTorque'  bp_nam='LoadPercent17'  breakpoint_data=LoadPercent17IdxArr  table_data=IndTorqueTbl  show_more=on  bp_data_type=Inherit from 'Breakpoint Data'  table_data_type=Inherit from 'Table Data'  storage=NonAdaptive  read_level=1  write_level=1  ovr_cals=on  use_help=on  help='Indicated Torque - From Load Percent'  bp_units='%'  table_units='N.m'  use_min_max=off  bp_min_val=-inf  bp_max_val=inf  min_val=-inf  max_val=inf  use_precision=off  use_breakpoint=off  b_precision=''  b_gain=1  b_offset=0  b_exp=1  use_table=off  t_precision=''  t_gain=1  t_offset=0  t_exp=1  use_links=on  input_name='LoadPercent'  output_name=''  use_mototune_group=on  mototune_group=lookup_group(gcb)
  motohawk_table_1d1 : MotoHawk_lib/Lookup Tables/motohawk_table_1d  nam='LoadPercent'  bp_nam='APC17'  breakpoint_data=APC17IdxArr  table_data=LoadPercentTbl  show_more=on  bp_data_type=Inherit from 'Breakpoint Data'  table_data_type=Inherit from 'Table Data'  storage=NonAdaptive  read_level=1  write_level=1  ovr_cals=on  use_help=on  help='Load Percent - From APC'  bp_units='mg'  table_units='%'  use_min_max=off  bp_min_val=-inf  bp_max_val=inf  min_val=-inf  max_val=inf  use_precision=off  use_breakpoint=off  b_precision=''  b_gain=1  b_offset=0  b_exp=1  use_table=off  t_precision=''  t_gain=1  t_offset=0  t_exp=1  use_links=on  input_name='APC'  output_name=''  use_mototune_group=on  mototune_group=lookup_group(gcb)
  APC [mg] : Outport
  Load [%] : Outport  Port=2
  IndTorque [N.m] : Outport  Port=3
  IndPower (kW) : Outport  Port=4
  IndWork (kJ) : Outport  Port=5
  wires:
  MAF [g/s]/1 -> Air Per Cylinder Calculation/1  "MAF"
  RPM/1 -> Air Per Cylinder Calculation/2, Calculate Power and Work/2(RPM)  "RPM"
  motohawk_table_1d/1 -> IndTorque [N.m]/1, Calculate Power and Work/1(IndTorque (N*m))  "IndTorque"
  Air Per Cylinder Calculation/1 -> motohawk_table_1d1/1, APC [mg]/1, motohawk_probe/1  "APC"
  motohawk_table_1d1/1 -> Load [%]/1, motohawk_table_1d/1  "Load"
  Calculate Power and Work/1(IndPower (kW)) -> IndPower (kW)/1  "IndPower"
  Calculate Power and Work/2(IndWork (kJ)) -> IndWork (kJ)/1  "IndWork"
  EventsPerRev/1 -> Air Per Cylinder Calculation/3

== system motohawk_engine_motoshare_lib/Mass Flow to Charge Mass Transform ==
  dm/dt [g/s] : Inport
  RPM : Inport  Port=2
  EventsPerRev : Inport  Port=3
  Data Type Conversion : DataTypeConversion  SaturateOnIntegerOverflow=on  RndMeth=Zero
  "Multiply and Divide, avoiding divde by zero" : Subsystem  TreatAsAtomicUnit=on
  NonZero RPM : motohawk_control_primitives_lib/CompareTo  op=~=  val=0
  Units Equivalency Factor : Constant  Value=60000
  m [mg] : Outport
  wires:
  RPM/1 -> NonZero RPM/1, "Multiply and Divide, avoiding divde by zero"/3(Divide1)
  NonZero RPM/1 -> "Multiply and Divide, avoiding divde by zero"/Enable
  Data Type Conversion/1 -> "Multiply and Divide, avoiding divde by zero"/4(Divide2)
  EventsPerRev/1 -> Data Type Conversion/1
  "Multiply and Divide, avoiding divde by zero"/1(" ") -> m [mg]/1
  Units Equivalency Factor/1 -> "Multiply and Divide, avoiding divde by zero"/2("X2 ")
  dm/dt [g/s]/1 -> "Multiply and Divide, avoiding divde by zero"/1(X1)

== system motohawk_engine_motoshare_lib/Model Fuel Puddle Mass ==
  DesFuelRate [g/s] : Inport
  MAF [g/s] : Inport  Port=2
  MAP [kPa] : Inport  Port=3
  ECT [degC] : Inport  Port=4
  IAT [degC] : Inport  Port=5
  Enabled Tau-X Algorithm : Subsystem
  If : If  Orientation=down  IfExpression=u1
  Merge : Merge
  Pass-Through : Subsystem
  motohawk_TitleBlock : Subsystem  mask{BlockType_='Mototron_Title_Block', ttl=[txtTitle '\newline\rmPer-Cylinder Transient Fueling Model\newlineSchedule Tau and X parameters on RPM and load'], im=mh.jpg}
      mask prompts: ttl "Description"; im "Image FIle"
      mask init:
      | set_param(gcb,'BlockType_','''Mototron_Title_Block''')
      | set_param(gcb,'MaskVisibilityString','off,on,on');
      mask Display:
      | image(imread(im),[0.31 0.66 0.31 0.35])
      | 
      | plot([0 0 1 1 0],[0 1 1 0 0])
      | plot([.3 1],[0.65 0.65])
      | plot([.3 .3],[0.1 1.0])
      | plot([0 1],[0.1 0.1])
      | plot([0.91 0.91],[0 0.1])
      | text(1,1,'\fontsize{22}\it\fontname{Arial Black}MotoTron Corporation \fontname{Arial}\fontsize{10}\newline505 Marion Road, Oshkosh, WI, 54901\newlinewww.mototron.com (734) 822-7700','verticalAlignment','Top','horizontalAlignment','Right','texmode','on')
      | text(0.01,1,['\fontsize{14}\it\bfPROPRIETARY\newlineAND CONFIDENTIAL\newline\fontsize{10}
      | THE INFORMATION CONTAINED IN THIS\newline
      | DRAWING IS THE SOLE PROPERTY OF\newline
      | MOTOTRON.  ANY REPRODUCTION IN\newline
      | PART OR AS A WHOLE WITHOUT THE\newline
      | WRITTEN PERMISSION OF MOTOTRON\newline
      | IS PROHIBITED.\fontsize{16}\rm\copyright\rm\fontsize{10} 2004' ],'verticalAlignment','Top','horizontalAlignment','Left','texmode','on')
      | 
      | text(0.9,0,['\fontsize{11}\bfPath: \rm' strrep(motohawk_vardec_path(gcb),'_','\_')],'verticalAlignment','Bottom','horizontalAlignment','Right','texmode','on')
      | text(0.31,0.65,['\fontsize{10}\bfDescription:'],'verticalAlignment','Top','horizontalAlignment','Left','texmode','on')
      | 
      | text(0.31,0.55,['\fontsize{14}\bf' ttl],'verticalAlignment','Top','horizontalAlignment','Left','texmode','on')
      | text(0.99,0,['\fontsize{11}\bfREV: \rm' motohawk_build_version],'verticalAlignment','Bottom','horizontalAlignment','Right','texmode','on')
  motohawk_calibration1 : MotoHawk_lib/Calibration & Probing Blocks/motohawk_calibration  nam='TransientFuelEnable'  val=0  storage=Calibration  show_more=on  name_source=Use Parameter  data_type=boolean  read_level=1  write_level=1  ovr_cals=on  view_as=Enumeration  enum_struct={'Disabled', 'Enabled'}  vector_style=Wide Row  use_help_units=on  help='Enable Tau-X transient fuel algorithm'  units=''  use_header_enum=off  row_header_enum={}  col_header_enum={}  use_min_max=off  min_val=-inf  max_val=inf  use_precision=off  precision=''  gain=1  offset=0  exp=1  use_mototune_group=on  mototune_group=group_cal
  FuelRate [g/s] : Outport
  wires:
  DesFuelRate [g/s]/1 -> Enabled Tau-X Algorithm/5(Fdes [g/s]), Pass-Through/1(Fdes [g/s])
  MAP [kPa]/1 -> Enabled Tau-X Algorithm/4(MAP [kPa])
  MAF [g/s]/1 -> Enabled Tau-X Algorithm/1(MAF [g/s])
  ECT [degC]/1 -> Enabled Tau-X Algorithm/3(ECT [degC])
  IAT [degC]/1 -> Enabled Tau-X Algorithm/2(IAT [degC])
  motohawk_calibration1/1 -> If/1
  If/1 -> Enabled Tau-X Algorithm/Action
  If/2 -> Pass-Through/Action
  Enabled Tau-X Algorithm/1(Finj [g/s]) -> Merge/1
  Pass-Through/1(Finj [g/s]) -> Merge/2
  Merge/1 -> FuelRate [g/s]/1
